simulink model "taska"  (R2022a)
settings: Solver=VariableStepAuto  StartTime=0.0  StopTime=10.0  RelTol=1e-3  EnableMultiTasking=on
settings Model: Creator=DSP AND COMM LAB  LastModifiedBy=Zonularity
settings SolverCC: AlgebraicLoopSolver=TrustRegion
settings DataIOCC: ReturnWorkspaceOutputs=off
settings OptimizationCC: LifeSpan=inf
settings DebuggingCC: UnconnectedInputMsg=warning  UnconnectedOutputMsg=warning  UnconnectedLineMsg=warning  SFUnexpectedBacktrackingDiag=warning  SFNoUnconditionalDefaultTransitionDiag=warning  SFMachineParentedDataDiag=warning  ArithmeticOperatorsInVariantConditions=warning
settings SFSimCC: SimUseLocalCustomCode=off  CustomCodeUndefinedFunction=UseInterfaceOnly
settings RTWCC: RTWUseLocalCustomCode=off
settings CodeAppCC: StateflowObjectComments=on
settings GRTTargetCC: TargetLangStandard=C89/C90 (ANSI)
settings ConfigComp: CovMetricSettings=dw  CovSaveCumulativeToWorkspaceVar=on  CovSaveSingleToWorkspaceVar=on  CovExternalEMLEnable=off

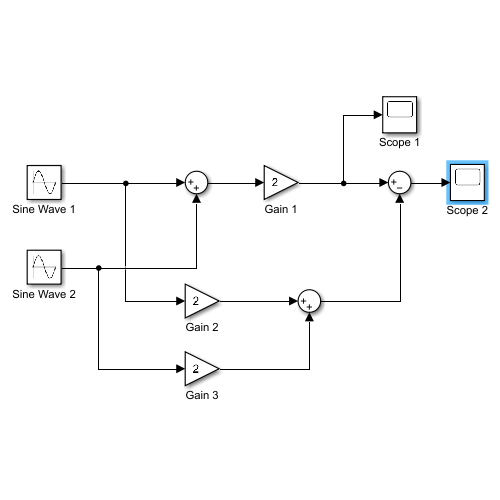
[thumbnail: Simulink's stored preview of the top-level diagram]
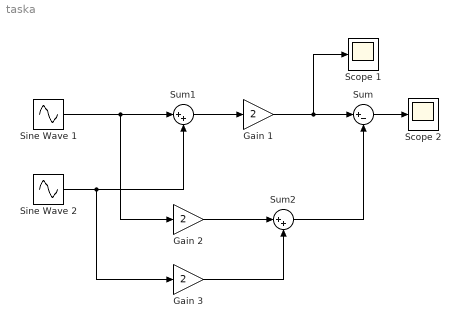
== system taska ==
  Gain 1 : Gain  Gain=2
  Gain 2 : Gain  Gain=2
  Gain 3 : Gain  Gain=2
  Scope 1 : Scope
  Scope 2 : Scope
  Sine Wave 1 : Sin  Frequency=2  SampleTime=0
  Sine Wave 2 : Sin  SampleTime=0
  Sum : Sum  Inputs=|+-
  Sum1 : Sum  Inputs=|++
  Sum2 : Sum  Inputs=|++
  wires:
  Sine Wave 1/1 -> Sum1/1, Gain 2/1
  Gain 1/1 -> Sum/1, Scope 1/1
  Sum/1 -> Scope 2/1
  Gain 2/1 -> Sum2/1
  Sum2/1 -> Sum/2
  Sine Wave 2/1 -> Gain 3/1, Sum1/2
  Sum1/1 -> Gain 1/1
  Gain 3/1 -> Sum2/2
